simulink model "controller"  (Simulink 8.0)
settings: Solver=FixedStepDiscrete  StartTime=0.0  StopTime=inf  FixedStep=Ts  RelTol=1e-3
InitFcn:
  | initRov14;
values from neighbouring files (symbols this model uses):
  fake = eye(25)    [initRov14.m]
  k = [  10    0.1   2 ... (first row only)    [initRov14.m]    (also in initSharedMem.m = [ 20    5   15)
undefined symbols (not defined in the file or in its folder): DiscIntNeverNeededParam
libraries: WBCLibrary x19, simulink x2, dspsigops x2
settings Model: Creator=daniele  LastModifiedBy=daniele
settings DebuggingCC: FcnCallInpInsideContextMsg=EnableAllAsWarning
settings GRTTargetCC: CombineOutputUpdateFcns=off  GRTInterface=on

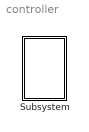
== system controller ==
  Subsystem : Subsystem  mask{robotName='icub', Ts=0.01, localName='dynamicBalancing'}
      mask prompts: robotName "robot name"; localName "module name"

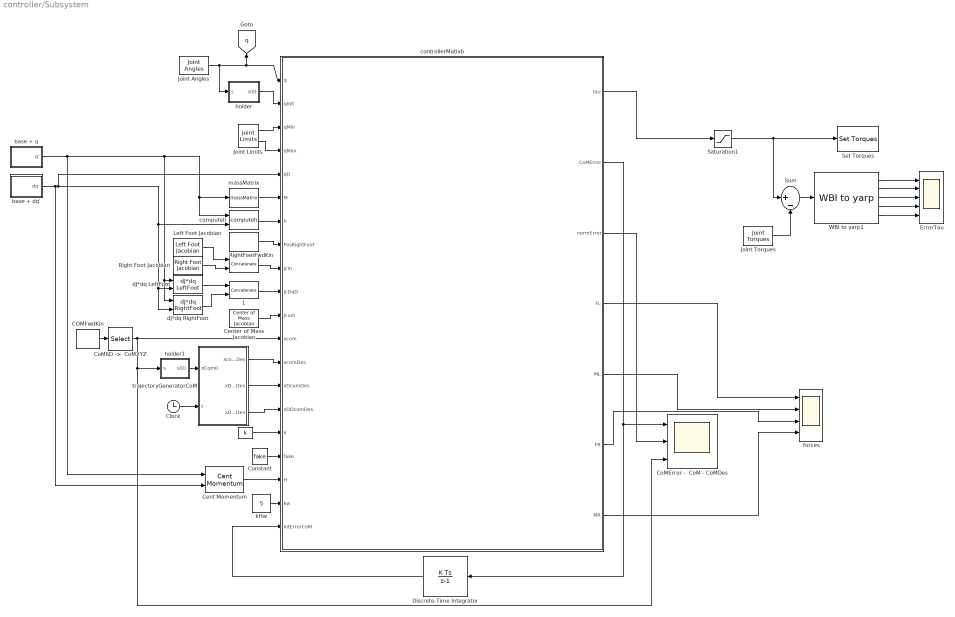
== system controller/Subsystem ==
  "    " : Constant  Value=k
  " " : Concatenate  Mode=Multidimensional array
  " 1" : Concatenate  Mode=Multidimensional array
  "COMFwdKin " : WBCLibrary/wholeBodyModel/Forward Kinematics/COMFwdKin   robotName=robotName  localName=localName
  Cent Momentum : WBCLibrary/wholeBodyModel/Dynamics/Cent Momentum  robotName=robotName  localName=localName
  Center of Mass Jacobian : WBCLibrary/wholeBodyModel/Jacobians/Center of Mass Jacobian  robotName=robotName  localName=localName
  Clock : Clock
  "CoM6D ->  CoMXYZ" : Selector  InputPortWidth=7  IndexOptions=Index vector (dialog)  Indices=[1 2 3]  OutputSizes=1
  "CoMError -  CoM - CoMDes " : Scope  NumInputPorts=3
      settings: TimeRange=70  YMin=-0.2~0.0175~-0.15  YMax=0.15~0.0525~0.55  SaveName=ScopeData6
  Constant : Constant  Value=fake
  Discrete-Time Integrator : DiscreteIntegrator  SampleTime=Ts  ICPrevOutput=DiscIntNeverNeededParam  ICPrevScaledInput=DiscIntNeverNeededParam
  ErrorTau : Scope  NumInputPorts=5
      settings: YMin=-12~-5~-5~-5~-5  YMax=12~5~5~5~5
  Joint Angles : WBCLibrary/wholeBodyStates/Joint Angles  robotName=robotName  localName=localName
  Joint Limits : WBCLibrary/wholeBodyModel/Joint Limits  robotName=robotName  localName=localName
  Joint Torques : WBCLibrary/wholeBodyStates/Joint Torques  robotName=robotName  localName=localName
  Left Foot Jacobian : WBCLibrary/wholeBodyModel/Jacobians/Left Foot Jacobian  robotName=robotName  localName=localName
  Right Foot Jacobian : WBCLibrary/wholeBodyModel/Jacobians/Right Foot Jacobian  robotName=robotName  localName=localName
  RightFootFwdKin : WBCLibrary/wholeBodyModel/Forward Kinematics/RightFootFwdKin  robotName=robotName  localName=localName
  Saturation1 : Saturate  UpperLimit=12  LowerLimit=-12  SampleTime=Ts
  Set Torques : WBCLibrary/wholeBodyActuators/Set Torques  val=6  robotName=robotName  localName=localName
  Sum : Sum  Inputs=|+-
  WBI to yarp1 : WBCLibrary/Utilities/WBI to yarp
  base + dq' : Subsystem
  base + q : Subsystem
  computeh : WBCLibrary/wholeBodyModel/Dynamics/computeh  val=7  robotname=robotName  localname=localName
  controllerMatlab : MATLAB Function  TreatAsAtomicUnit=on
  dJ*dq LeftFoot : WBCLibrary/wholeBodyModel/Dynamics/dJ*dq LeftFoot  val=9  robotName=robotName  localName=localName
  dJ*dq RightFoot : WBCLibrary/wholeBodyModel/Dynamics/dJ*dq RightFoot  val=9  robotName=robotName  localName=localName
  "forces " : Scope  NumInputPorts=4
      settings: ShowLegends=on  YMin=-12~-5~-5~-5  YMax=12~5~5~5
  holder : Subsystem
  holder1 : Subsystem
  kHw : Constant  Value=5
  massMatrix : WBCLibrary/wholeBodyModel/Dynamics/massMatrix  val=8  robotname=robotName  localname=localName
  trajectoryGeneratorCoM : MATLAB Function  TreatAsAtomicUnit=on
  tag scope: q=global
  wires:
  computeh/1 -> controllerMatlab/7(h)
  massMatrix/1 -> controllerMatlab/6(M)
  Joint Angles/1 -> holder/1(s), [q], controllerMatlab/1(q)
  Center of Mass Jacobian/1 -> controllerMatlab/11(Jcom)
  "    "/1 -> controllerMatlab/16(k)
  Left Foot Jacobian/1 -> " "/1
  Right Foot Jacobian/1 -> " "/2
  trajectoryGeneratorCoM/1(xcomDes) -> controllerMatlab/13(xcomDes)
  trajectoryGeneratorCoM/2(xDcomDes) -> controllerMatlab/14(xDcomDes)
  trajectoryGeneratorCoM/3(xDDcomDes) -> controllerMatlab/15(xDDcomDes)
  Clock/1 -> trajectoryGeneratorCoM/2(t)
  holder1/1(s(0)) -> trajectoryGeneratorCoM/1(xCom0)
  dJ*dq LeftFoot/1 -> " 1"/1
  dJ*dq RightFoot/1 -> " 1"/2
  "COMFwdKin "/1 -> "CoM6D ->  CoMXYZ"/1
  "CoM6D ->  CoMXYZ"/1 -> holder1/1(s), "CoMError -  CoM - CoMDes "/3, controllerMatlab/12(xcom)
  holder/1(s(0)) -> controllerMatlab/2(qInit)
  RightFootFwdKin/1 -> controllerMatlab/8(PosRightFoot)
  controllerMatlab/2(CoMError) -> Discrete-Time Integrator/1, "CoMError -  CoM - CoMDes "/1
  Discrete-Time Integrator/1 -> controllerMatlab/20(IntErrorCoM)
  base + q/1(q') -> computeh/1, massMatrix/1, dJ*dq RightFoot/1, dJ*dq LeftFoot/1, Cent Momentum/1
  base + dq'/1(dq') -> controllerMatlab/5(qD), computeh/2, dJ*dq RightFoot/2, dJ*dq LeftFoot/2, Cent Momentum/2
  Cent Momentum/1 -> controllerMatlab/18(H)
  kHw/1 -> controllerMatlab/19(kw)
  Constant/1 -> controllerMatlab/17(fake)
  controllerMatlab/3(normError) -> "CoMError -  CoM - CoMDes "/2
  " 1"/1 -> controllerMatlab/10(JcDqD)
  " "/1 -> controllerMatlab/9(JcIn)
  Joint Torques/1 -> Sum/2
  Saturation1/1 -> Sum/1, Set Torques/1
  WBI to yarp1/1 -> ErrorTau/1
  WBI to yarp1/2 -> ErrorTau/2
  WBI to yarp1/3 -> ErrorTau/3
  WBI to yarp1/4 -> ErrorTau/4
  Sum/1 -> WBI to yarp1/1
  WBI to yarp1/5 -> ErrorTau/5
  controllerMatlab/4(FL) -> "forces "/1
  controllerMatlab/5(ML) -> "forces "/2
  controllerMatlab/6(FR) -> "forces "/3
  controllerMatlab/7(MR) -> "forces "/4
  controllerMatlab/1(tau) -> Saturation1/1
  Joint Limits/1 -> controllerMatlab/3(qMin)
  Joint Limits/2 -> controllerMatlab/4(qMax)

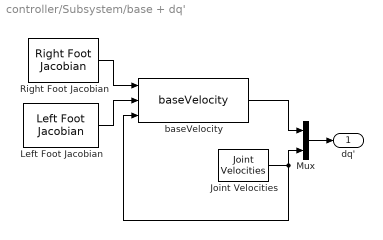
== system controller/Subsystem/base + dq' ==
  Joint Velocities : WBCLibrary/wholeBodyStates/Joint Velocities  robotName=robotName  localName=localName
  Left Foot Jacobian : WBCLibrary/wholeBodyModel/Jacobians/Left Foot Jacobian  robotName=robotName  localName=localName
  Mux : Mux  Inputs=2
  Right Foot Jacobian : WBCLibrary/wholeBodyModel/Jacobians/Right Foot Jacobian  robotName=robotName  localName=localName
  baseVelocity : WBCLibrary/Utilities/baseVelocity
  dq' : Outport
  wires:
  Left Foot Jacobian/1 -> baseVelocity/2
  Right Foot Jacobian/1 -> baseVelocity/1
  baseVelocity/1 -> Mux/1
  Joint Velocities/1 -> baseVelocity/3, Mux/2
  Mux/1 -> dq'/1

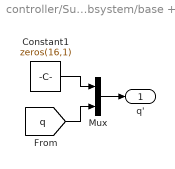
== system controller/Subsystem/base + q ==
  Constant1 : Constant  Value=zeros(16,1)
  Mux : Mux  Inputs=2
  q' : Outport
  wires:
  Mux/1 -> q'/1
  [q] -> Mux/2
  Constant1/1 -> Mux/1

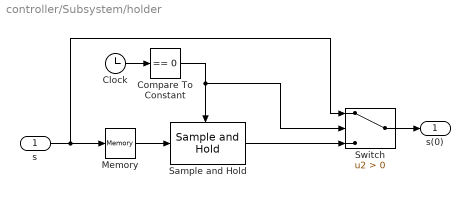
== system controller/Subsystem/holder ==
  s : Inport
  Clock : Clock
  Compare To Constant : simulink/Logic and Bit Operations/Compare To Constant  relop===  const=0  OutDataTypeStr=boolean
  Memory : Memory
  Sample and Hold : dspsigops/Sample and Hold  trig=Falling edge  initCond=0  latchinput=off
  Switch : Switch  Criteria=u2 > Threshold
  s(0) : Outport
  wires:
  s/1 -> Switch/1, Memory/1
  Clock/1 -> Compare To Constant/1
  Compare To Constant/1 -> Sample and Hold/Trigger, Switch/2
  Sample and Hold/1 -> Switch/3
  Switch/1 -> s(0)/1
  Memory/1 -> Sample and Hold/1

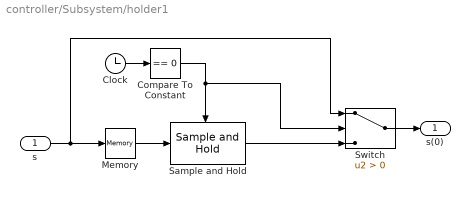
== system controller/Subsystem/holder1 ==
  s : Inport
  Clock : Clock
  Compare To Constant : simulink/Logic and Bit Operations/Compare To Constant  relop===  const=0  OutDataTypeStr=boolean
  Memory : Memory
  Sample and Hold : dspsigops/Sample and Hold  trig=Falling edge  initCond=0  latchinput=off
  Switch : Switch  Criteria=u2 > Threshold
  s(0) : Outport
  wires:
  s/1 -> Switch/1, Memory/1
  Clock/1 -> Compare To Constant/1
  Compare To Constant/1 -> Sample and Hold/Trigger, Switch/2
  Sample and Hold/1 -> Switch/3
  Switch/1 -> s(0)/1
  Memory/1 -> Sample and Hold/1

== matlab function Subsystem/trajectoryGeneratorCoM ==
  data: xcomDes output double; xDcomDes output double; xDDcomDes output double; xCom0 input double; t input double
function [xcomDes, xDcomDes, xDDcomDes] = fcn(xCom0,t)
%#codegen

e3 = [0;1;0];
A = 0.0;
f = 0.1;
t = t*0.8;
% xcomDes    = [xCom0(1:2); (1/A-1)*A*xCom0(3)] + A*xCom0(3)*cos(2*pi*f*t)*e3;
% xDcomDes   = -xCom0(3)*A*2*pi*f*sin(2*pi*f*t)*e3;
% xDDcomDes  = -xCom0(3)*A*(2*pi*f)^2*cos(2*pi*f*t)*e3;

xcomDes    = xCom0 + A*sin(2*pi*f*t)*e3;
xcomDes(1) =  xcomDes(1) + 0.03;
xDcomDes   =         A*2*pi*f*cos(2*pi*f*t)*e3;
xDDcomDes  =        -A*(2*pi*f)^2*sin(2*pi*f*t)*e3;

== matlab function Subsystem/controllerMatlab ==
  data: q input double; qInit input double; qMin input double; qMax input double; qD input double; M input double; h input double; PosRightFoot input double; JcIn input double; JcDqD input double; tau output double; Jcom input double; xcom input double; xcomDes input double; xDcomDes input double; xDDcomDes input double; k input double; fake input double; H input double; kw input double; CoMError output double; IntErrorCoM input double; normError output double; FL output double; ML output double; FR output double; MR output double
function [tau,CoMError,normError,FL,ML,FR,MR] = fcn(q,qInit,qMin,qMax, qD, M, h, PosRightFoot, JcIn, JcDqD, Jcom, xcom, xcomDes, xDcomDes, xDDcomDes, k, fake, H, kw,IntErrorCoM)
%#codegen

PINV_TOL = 1e-5;
g        = 9.81;

n = size(fake, 1);

DL = 25-n;            %DeltaIndexOnlyLegs

if DL ~= 0
   Jc = [JcIn(:,1:6),JcIn(:,7 + DL:end)]; 
else
   Jc = JcIn; 
end

m     = M(1,1);
Mb    = M(1:6,1:6);
MbInv = inv(Mb);
Mbj   = M(1:6,7 + DL :end); 
Mj    = M(7 + DL :end,7 + DL:end);
U     = [eye(6) , zeros(6,n)];
Jcb   = Jc*U';
SBar  = [  -MbInv*Mbj 
           eye(n)      ];
NjInv = Mj - Mbj'*MbInv*Mbj;

grav = [zeros(2,1);-m*g;zeros(3,1)];

JcSBar     = Jc*SBar;
JcSBarPinv = pinv(JcSBar, PINV_TOL);

% Definition of reference accelerations for CoM and Joints that ensure
% stabilization of desired trajectories xDcomDes and qDes 

xDcom      = Jcom(1:3,:)*qD;
xDDcomStar = xDDcomDes - k(1,1)*(xcom - xcomDes) - k(1,2)*IntErrorCoM - k(1,3)*(xDcom - xDcomDes)  ;
q_starIn   =           - kPost*(q - qInit)                            - k(2,3)*qD(7:end);
if DL ~= 0
   q_star = q_starIn(DL+1:end); 
else
   q_star = q_starIn;
    
end
Pr =  PosRightFoot(1:3) - xcom; % Application point of the contact force on the right foot w.r.t. CoM
A  = [ eye(3),   zeros(3),eye(3), zeros(3);
      -Sf(xcom),  eye(3), Sf(Pr), eye(3) ];

% The following expressions for Ic and IcD hold only if the control 
% objective is the stabilization of the CoM's position
% kw = 0.1;
hwDotDes = H(4:end);
hDotDes = [ m*xDDcomStar ;
            -kw*hwDotDes  ]; 

fd = pinv(A)*(hDotDes-grav);

LambdaStar = JcSBarPinv*(Jcb*MbInv*(h(1:6) - Jcb'*fd) - JcDqD);

NP0 = eye(n) - JcSBarPinv*JcSBar;

LambdaStar = LambdaStar + NP0 *( q_star - LambdaStar);

tauLegs = - JcSBar'*fd + NjInv*LambdaStar + SBar'*[h(1:6);h(DL + 7:end)];

if DL >= 1 
   tau = h(7:end) - k(3,1)*(q - qInit) - k(3,3)*qD(7:end);   
   tau(DL+1:end) = tauLegs;
else
    tau = tauLegs;
end

FL = fd(1:3);
ML = fd(4:6);
FR = fd(7:9);
MR = fd(10:12);

CoMError    = xcom - xcomDes;
normError   = norm(CoMError);
